simulink model "Circuit_tuner_model"  (R2022a)
settings: Solver=FixedStepAuto  StartTime=0.0  StopTime=.004  FixedStep=SampleTime  RelTol=1e-3
values from neighbouring files (symbols this model uses):
  Ad = sys_d_plasma.A    [All_injectors_LQG_bop_plasma_ss_model_code.m]    (also in All_injectors_LQG_bop_ss_model_code.m; All_injectors_LQG_continuous_time_code.m; All_injectors_LQG_plasma_7_15_24_code.m; All_injectors_LQG_plasma_ss_model_code.m)
  Amplitude = 600    [All_injectors_LQG_bop_plasma_ss_model_code.m]    (also in All_injectors_LQG_bop_ss_model_code.m; All_injectors_LQG_continuous_time_code.m; All_injectors_LQG_plasma_7_15_24_code.m; All_injectors_LQG_plasma_ss_model_code.m)
  Amplitude1 = 600    [All_injectors_vaccum.m]    (also in All_injectors_with_LQG_code.m; MPC_attempt.m; Plasma_ss_model.m; Use_for_freq_scan.m)
  Bd = sys_d_plasma.B    [All_injectors_LQG_bop_plasma_ss_model_code.m]    (also in All_injectors_LQG_bop_ss_model_code.m; All_injectors_LQG_continuous_time_code.m; All_injectors_LQG_plasma_7_15_24_code.m; All_injectors_LQG_plasma_ss_model_code.m)
  Cap = 96e-6    (= 9.6e-05)    [All_injectors_LQG_bop_ss_model_code.m]    (also in All_injectors_LQG_continuous_time_code.m; All_injectors_LQG_plasma_7_15_24_code.m; All_injectors_LQG_plasma_ss_model_code.m; All_injectors_vaccum.m)
  Cd = sys_d_plasma.C    [All_injectors_LQG_bop_plasma_ss_model_code.m]    (also in All_injectors_LQG_bop_ss_model_code.m; All_injectors_LQG_continuous_time_code.m; All_injectors_LQG_plasma_7_15_24_code.m; All_injectors_LQG_plasma_ss_model_code.m)
  Dd = sys_d_plasma.D    [All_injectors_LQG_bop_plasma_ss_model_code.m]    (also in All_injectors_LQG_bop_ss_model_code.m; All_injectors_LQG_continuous_time_code.m; All_injectors_LQG_plasma_7_15_24_code.m; All_injectors_LQG_plasma_ss_model_code.m)
  L1 = (9.78e-7)    (= 9.78e-07)    [All_injectors_LQG_bop_plasma_ss_model_code.m]    (also in All_injectors_LQG_bop_ss_model_code.m = 8.0141e-07; All_injectors_LQG_continuous_time_code.m = 8.0141e-07; All_injectors_LQG_plasma_7_15_24_code.m = 8.0141e-07; All_injectors_LQG_plasma_ss_model_code.m = 8.0141e-07)
  L2 = 2.0462e-6    (= 2.0462e-06)    [All_injectors_LQG_bop_ss_model_code.m]    (also in All_injectors_LQG_continuous_time_code.m; All_injectors_LQG_plasma_7_15_24_code.m; All_injectors_LQG_plasma_ss_model_code.m; All_injectors_vaccum.m)
  Lp = L2    (= 2.0462e-06)    [All_injectors_LQG_bop_ss_model_code.m]    (also in All_injectors_LQG_continuous_time_code.m; All_injectors_LQG_plasma_7_15_24_code.m; All_injectors_LQG_plasma_ss_model_code.m; Plasma_ss_model.m = 1.0231e-06)
  M = .161*L2    (= 3.294382e-07)    [All_injectors_LQG_bop_ss_model_code.m]    (also in All_injectors_LQG_continuous_time_code.m; All_injectors_LQG_plasma_7_15_24_code.m; All_injectors_LQG_plasma_ss_model_code.m; All_injectors_vaccum.m)
  Mw = .1346*L2    (= 2.7541852e-07)    [All_injectors_LQG_bop_ss_model_code.m]    (also in All_injectors_LQG_continuous_time_code.m; All_injectors_LQG_plasma_7_15_24_code.m; All_injectors_LQG_plasma_ss_model_code.m; All_injectors_vaccum.m)
  NoisePower = 0    [All_injectors_LQG_bop_plasma_ss_model_code.m]    (also in All_injectors_LQG_bop_ss_model_code.m = 0.0001; All_injectors_LQG_continuous_time_code.m = 0.0001; All_injectors_LQG_plasma_7_15_24_code.m; All_injectors_LQG_plasma_ss_model_code.m = 0.0001)
  R = 1    [All_injectors_LQG_bop_plasma_ss_model_code.m]    (also in All_injectors_LQG_bop_ss_model_code.m = diag(1*ones(1,num_inputs)); All_injectors_LQG_continuous_time_code.m = diag(1*ones(1,num_inputs)); All_injectors_LQG_plasma_7_15_24_code.m = diag(1*ones(1,num_inputs)); All_injectors_LQG_plasma_ss_model_code.m = diag(1*ones(1,num_inputs)))
  R1 = .0025    (= 0.0025)    [All_injectors_LQG_bop_ss_model_code.m]    (also in All_injectors_LQG_continuous_time_code.m; All_injectors_LQG_plasma_7_15_24_code.m; All_injectors_LQG_plasma_ss_model_code.m; All_injectors_vaccum.m)
  R2 = .005    (= 0.005)    [All_injectors_LQG_bop_ss_model_code.m]    (also in All_injectors_LQG_continuous_time_code.m; All_injectors_LQG_plasma_7_15_24_code.m; All_injectors_LQG_plasma_ss_model_code.m; All_injectors_vaccum.m)
  R3 = .005    (= 0.005)    [All_injectors_LQG_bop_ss_model_code.m]    (also in All_injectors_LQG_continuous_time_code.m; All_injectors_LQG_plasma_7_15_24_code.m; All_injectors_LQG_plasma_ss_model_code.m; All_injectors_vaccum.m)
  RunTime = .004    (= 0.004)    [All_injectors_LQG_bop_plasma_ss_model_code.m]    (also in All_injectors_LQG_bop_ss_model_code.m; All_injectors_LQG_continuous_time_code.m; All_injectors_LQG_plasma_7_15_24_code.m; All_injectors_LQG_plasma_ss_model_code.m)
  SampleTime = 1e-7    (= 1e-07)    [All_injectors_LQG_bop_plasma_ss_model_code.m]    (also in All_injectors_LQG_bop_ss_model_code.m; All_injectors_LQG_continuous_time_code.m; All_injectors_LQG_plasma_7_15_24_code.m; All_injectors_LQG_plasma_ss_model_code.m)
  voltage = Amplitude*sin(2*pi*Frequency*time)    [All_injectors_LQG_bop_plasma_ss_model_code.m]    (also in All_injectors_LQG_bop_ss_model_code.m; All_injectors_LQG_continuous_time_code.m; All_injectors_LQG_plasma_7_15_24_code.m; All_injectors_LQG_plasma_ss_model_code.m)
undefined symbols (not defined in the file or in its folder): Discrete, L1_V, Time
libraries: spsSeriesRLCBranchLib x49, simulink x22, spsCurrentMeasurementLib x20, spsVoltageMeasurementLib x14, spsDCVoltageSourceLib x12, spsFullBridgeMMCExternalDCLinksLib x9, spsPWMGeneratorMultilevelLib x9, spsParallelRLCBranchLib x6, ctrlSharedLib x5, spsMosfetLib x4, spsControlledVoltageSourceLib x1, spsMutualInductanceLib x1
(part 1 of 2)
settings Model: Creator=ducks  LastModifiedBy=ducks
settings DataIOCC: ExternalInput=[t,V]

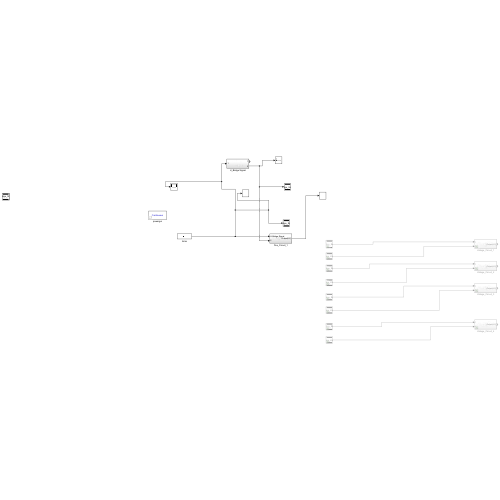
[thumbnail: Simulink's stored preview of the top-level diagram]
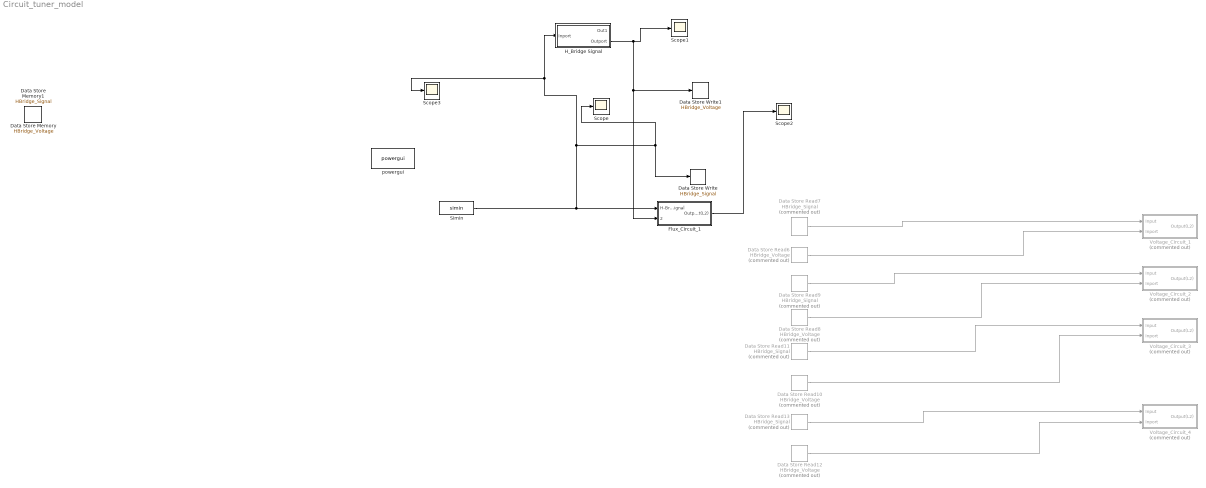
== system Circuit_tuner_model ==
  Data Store Read{6,8,10,12} (4 alike) : DataStoreRead  Commented=on  DataStoreName=HBridge_Voltage  IndexOptions=Index vector (dialog)  Indices=1  OutputSizes=1
  Data Store Read{7,9,11,13} (4 alike) : DataStoreRead  Commented=on  DataStoreName=HBridge_Signal  IndexOptions=Index vector (dialog)  Indices=1  OutputSizes=1
  Data Store Write : DataStoreWrite  DataStoreName=HBridge_Signal  IndexOptions=Index vector (dialog)  Indices=1  OutputSizes=1
  Data Store Write1 : DataStoreWrite  DataStoreName=HBridge_Voltage  IndexOptions=Index vector (dialog)  Indices=1  OutputSizes=1
  Data Store Memory : DataStoreMemory  DataStoreName=HBridge_Voltage  WriteAfterWriteMsg=warning  ShowAdditionalParam=off
  Data Store Memory1 : DataStoreMemory  DataStoreName=HBridge_Signal  WriteAfterWriteMsg=warning  ShowAdditionalParam=off
  Flux_Circuit_1 : Subsystem
  H_Bridge Signal : Subsystem
  Scope{,1..3} (4 alike) : Scope
  Simin : FromWorkspace  VariableName=simin
  Voltage_Circuit_1 : Subsystem  Commented=on
  Voltage_Circuit_2 : Subsystem  Commented=on
  Voltage_Circuit_3 : Subsystem  Commented=on
  Voltage_Circuit_4 : Subsystem  Commented=on
  powergui : spspowerguiLib/powergui  Priority=1  SimulationMode=Continuous  SampleTime=50e-6  frequency=60  Iterations=50  frequencyindice=0  Pbase=100e6  ErrMax=1e-4  UnitsV=kV  UnitsW=MW  buscounter=0  FunctionMessages=off  echomessages=off  EnableUseOfTLC=off  CurrentSourceSwitches=off  DisableSnubberDevices=off  DisableRonSwitches=off  DisableVfSwitches=off  DisplayEquations=off  AutomaticDiscreteSolvers=off  SolverType=Tustin/Backward Euler (TBE)  Interpol=off  ExternalGateDelay=off  methode=off  Ts=100  x0status=blocks  SPID=on  SwTol=0  HookPort=off  NonlinearTolerance=1e-4  nMaxIteration=100  ContinueOnMaxIteration=off  RestoreLinks=warning  ResistiveCurrentMeasurement=off  Frange=[0:2:500]  Ylog=off  Xlog=on  ShowGrid=off  save=off  variable=ZData  structure=0  ZoomFFT=off  StartTime=0.0  cycles=1  DisplayStyle=1  fundamental=60  FreqAxis=off  MaxFrequency=1000  frequencyindicesteady=1  RmsSteady=1  display=off
  wires:
  Flux_Circuit_1/1(Output(L2)) -> Scope2/1
  H_Bridge Signal/2(Outport) -> Data Store Write1/1, Flux_Circuit_1/2(2), Scope1/1
  Simin/1 -> Scope3/1, H_Bridge Signal/1(Inport), Scope/1, Data Store Write/1, Flux_Circuit_1/1(H-Bridge Signal)
  Data Store Read6/1 -> Voltage_Circuit_1/2(Inport)
  Data Store Read7/1 -> Voltage_Circuit_1/1(Input)
  Data Store Read8/1 -> Voltage_Circuit_2/2(Inport)
  Data Store Read9/1 -> Voltage_Circuit_2/1(Input)
  Data Store Read10/1 -> Voltage_Circuit_3/2(Inport)
  Data Store Read11/1 -> Voltage_Circuit_3/1(Input)
  Data Store Read12/1 -> Voltage_Circuit_4/2(Inport)
  Data Store Read13/1 -> Voltage_Circuit_4/1(Input)

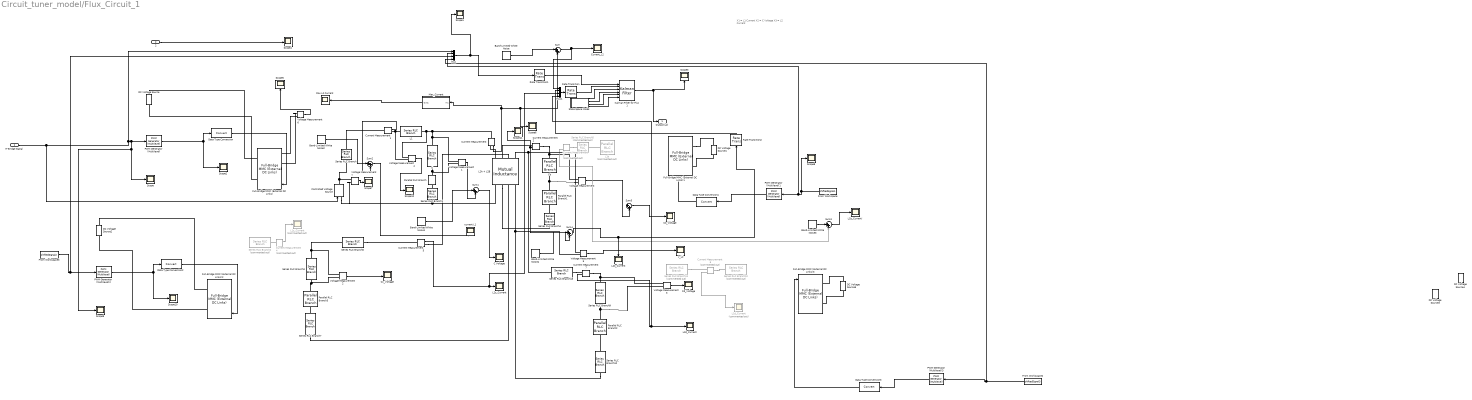
== system Circuit_tuner_model/Flux_Circuit_1 ==
  note: X1 = L1 Current
      | X2 = C Voltage
      | X3 = L2 Current
  H-Bridge Signal : Inport
  2 : Inport  Port=2
  Band-Limited White Noise{,2..4} (4 alike) : simulink/Sources/Band-Limited White Noise  Cov=NoisePower  Ts=SampleTime  seed=[23341]
  Band-Limited White Noise1 : simulink/Sources/Band-Limited White Noise  Cov=NoisePower/5  Ts=SampleTime  seed=[23341]
  C : spsSeriesRLCBranchLib/Series RLC Branch  LConnTagsString=__new0  RConnTagsString=__new0  BranchType=C  Resistance=1  Inductance=1e-3  SetiL0=off  InitialCurrent=0  Capacitance=Cap  Setx0=off  InitialVoltage=0  Measurements=None
  C Voltage : Scope
  Cb : spsParallelRLCBranchLib/Parallel RLC Branch  LConnTagsString=a  RConnTagsString=__new0  BranchType=C  Resistance=1  Inductance=1e-3  SetiL0=off  InitialCurrent=0  Capacitance=Cap  Setx0=off  InitialVoltage=0  Measurements=None
  Cb_Voltage : Scope
  Cc_Voltage : Scope
  Cd_Voltage : Scope
  Controlled Voltage Source : spsControlledVoltageSourceLib/Controlled Voltage Source  Initialize=on  Source_Type=AC  Amplitude=0  Phase=0  Frequency=0  Measurements=None
  Current Measurement{,1..2,5,7} (5 alike) : spsCurrentMeasurementLib/Current Measurement  PhasorSimulation=off  OutputType=Complex  PSBequivalent=0
  Current Measurement3 : spsCurrentMeasurementLib/Current Measurement  Commented=on  PhasorSimulation=off  OutputType=Complex  PSBequivalent=0
  Current Measurement4 : spsCurrentMeasurementLib/Current Measurement  Commented=on  PhasorSimulation=off  OutputType=Complex  PSBequivalent=0
  Current Measurement6 : spsCurrentMeasurementLib/Current Measurement  Commented=on  PhasorSimulation=off  OutputType=Complex  PSBequivalent=0
  Current_L2 : Scope
  DC Voltage Source : spsDCVoltageSourceLib/DC Voltage Source  Amplitude=Amplitude  Measurements=None
  DC Voltage Source1 : spsDCVoltageSourceLib/DC Voltage Source  Amplitude=Amplitude1  Measurements=None
  DC Voltage Source2 : spsDCVoltageSourceLib/DC Voltage Source  Amplitude=Amplitude1  Measurements=None
  DC Voltage Source3 : spsDCVoltageSourceLib/DC Voltage Source  Amplitude=Amplitude  Measurements=None
  DC Voltage Source4 : spsDCVoltageSourceLib/DC Voltage Source  Amplitude=Amplitude  Measurements=None
  DC Voltage Source5 : spsDCVoltageSourceLib/DC Voltage Source  Amplitude=Amplitude1  Measurements=None
  Data Type Conversion{,1..3} (4 alike) : DataTypeConversion  SaturateOnIntegerOverflow=off  RndMeth=Floor
  From Workspace : FromWorkspace  VariableName=shiftedSignal1
  From Workspace2 : FromWorkspace  VariableName=shiftedSignal3
  From Workspace3 : FromWorkspace  VariableName=shiftedSignal2
  Full-Bridge MMC (External DC Links){,1..3} (4 alike) : spsFullBridgeMMCExternalDCLinksLib/Full-Bridge MMC (External DC Links)  ModelType=Switching devices  n=1  Ron=1e-3  Rs=1e6  Cs=inf  Ron_Diode=1e-3  Rs_Diode=1e6  Cs_Diode=inf  Vf_Diode=1e-3  Rs_CurrentSource=inf  Ts=1e-6
      settings: SourceProductBaseCode=PS
  Kalman Filter for Flux 1 : ctrlSharedLib/Kalman Filter  TimeDomain=Discrete-Time  UseCurrentEstimator=on  ModelSource=Input port  ModelSourceVariable=sys_d  A=Ad  B=Bd  C=Cd  D=Dd  NumberOfStates=12  NumberOfInputs=4  NumberOfOutputs=4  InitialEstimateSource=Dialog  X0=voltage(1)  P0=10  UseK=off  UseGH=off  NumberOfProcessNoiseInputs=1  G=G  TimeInvariantG=on  H=0  TimeInvariantH=on  Q=Q  TimeInvariantQ=on  R=R  TimeInvariantR=on  N=0  TimeInvariantN=on  AddInputPort=on  AddEnablePort=off  OutputEstimatedY=off  OutputP=off  Ts=SampleTime
  L1 : spsSeriesRLCBranchLib/Series RLC Branch  LConnTagsString=__new0  RConnTagsString=__new0  BranchType=L  Resistance=1  Inductance=L1  SetiL0=off  InitialCurrent=0  Capacitance=0  Setx0=off  InitialVoltage=0  Measurements=None
  L1b : spsParallelRLCBranchLib/Parallel RLC Branch  Commented=on  LConnTagsString=a  RConnTagsString=__new0  BranchType=L  Resistance=1  Inductance=L1  SetiL0=off  InitialCurrent=0  Capacitance=1e-6  Setx0=off  InitialVoltage=0  Measurements=None
  L1b_Current' : Scope
  L1c_Current : Scope  Commented=on
  L1d_Current : Scope  Commented=on
  L2A + L2B : spsMutualInductanceLib/Mutual Inductance  LConnTagsString=a|b|c|L4  RConnTagsString=A|B|C|R4  TypeOfMutual=Generalized mutual inductance  NumberOfWindings=4  SelfImpedance1=[R3 L2]  SelfImpedance2=[R3 L2]  ThreeWindings=on  SelfImpedance3=[ 1.1 1.1e-03]  MutualImpedance=[R3/2 L2/2]  InductanceMatrix=[L2 M M Mw; M L2 Mw M; M Mw L2 M; Mw M M L2;]  ResistanceMatrix=[R3 0 0 0; 0 R3 0 0; 0 0 R3 0; 0 0 0 R3;]  Measurements=Winding voltages and currents
      settings: SourceProductBaseCode=PS
  L2b_Current : Scope
  L2c_Current : Scope
  L2d_Current : Scope
  Max L2 Current : Scope
  Max_Current : Subsystem
  Mux : Mux
  Mux1 : Mux
  PWM Generator (Multilevel){,1..3} (4 alike) : spsPWMGeneratorMultilevelLib/PWM Generator (Multilevel)  BridgeType=Full-bridge  NumberOfBridges=1  Fc=1e3  Ts=0  ShowCarriersOutport=off
      settings: SourceProductBaseCode=PS
  Parallel RLC Branch{,1..3} (4 alike) : spsParallelRLCBranchLib/Parallel RLC Branch  LConnTagsString=a  RConnTagsString=__new0  BranchType=L  Resistance=1  Inductance=100e-9  SetiL0=off  InitialCurrent=0  Capacitance=1e-6  Setx0=off  InitialVoltage=0  Measurements=None
  Rate Transition : RateTransition
  Rate Transition1 : RateTransition
  Rate Transition2 : RateTransition
  Scope{,1..12} (13 alike) : Scope
  Series RLC Branch : spsSeriesRLCBranchLib/Series RLC Branch  LConnTagsString=__new0  RConnTagsString=__new0  BranchType=R  Resistance=R1  Inductance=1e-3  SetiL0=off  InitialCurrent=0  Capacitance=1e-6  Setx0=off  InitialVoltage=0  Measurements=None
  Series RLC Branch{1,4,7,12} (4 alike) : spsSeriesRLCBranchLib/Series RLC Branch  LConnTagsString=__new0  RConnTagsString=__new0  BranchType=R  Resistance=R2  Inductance=1e-3  SetiL0=off  InitialCurrent=0  Capacitance=1e-6  Setx0=off  InitialVoltage=0  Measurements=None
  Series RLC Branch10 : spsSeriesRLCBranchLib/Series RLC Branch  Commented=on  LConnTagsString=__new0  RConnTagsString=__new0  BranchType=L  Resistance=1  Inductance=L1  SetiL0=off  InitialCurrent=0  Capacitance=1e-6  Setx0=off  InitialVoltage=0  Measurements=None
  Series RLC Branch11 : spsSeriesRLCBranchLib/Series RLC Branch  Commented=on  LConnTagsString=__new0  RConnTagsString=__new0  BranchType=R  Resistance=R1  Inductance=1e-3  SetiL0=off  InitialCurrent=0  Capacitance=1e-6  Setx0=off  InitialVoltage=0  Measurements=None
  Series RLC Branch13 : spsSeriesRLCBranchLib/Series RLC Branch  LConnTagsString=__new0  RConnTagsString=__new0  BranchType=R  Resistance=R3  Inductance=1e-3  SetiL0=off  InitialCurrent=0  Capacitance=1e-6  Setx0=off  InitialVoltage=0  Measurements=None
  Series RLC Branch2 : spsSeriesRLCBranchLib/Series RLC Branch  Commented=on  LConnTagsString=__new0  RConnTagsString=__new0  BranchType=L  Resistance=1  Inductance=L1  SetiL0=off  InitialCurrent=0  Capacitance=1e-6  Setx0=off  InitialVoltage=0  Measurements=None
  Series RLC Branch3 : spsSeriesRLCBranchLib/Series RLC Branch  LConnTagsString=__new0  RConnTagsString=__new0  BranchType=C  Resistance=1  Inductance=L2  SetiL0=off  InitialCurrent=0  Capacitance=Cap  Setx0=off  InitialVoltage=0  Measurements=None
  Series RLC Branch5 : spsSeriesRLCBranchLib/Series RLC Branch  Commented=on  LConnTagsString=__new0  RConnTagsString=__new0  BranchType=R  Resistance=R1  Inductance=1e-3  SetiL0=off  InitialCurrent=0  Capacitance=1e-6  Setx0=off  InitialVoltage=0  Measurements=None
  Series RLC Branch6 : spsSeriesRLCBranchLib/Series RLC Branch  LConnTagsString=__new0  RConnTagsString=__new0  BranchType=R  Resistance=R3  Inductance=1e-3  SetiL0=off  InitialCurrent=0  Capacitance=1e-6  Setx0=off  InitialVoltage=0  Measurements=None
  Series RLC Branch9 : spsSeriesRLCBranchLib/Series RLC Branch  LConnTagsString=__new0  RConnTagsString=__new0  BranchType=C  Resistance=1  Inductance=1e-3  SetiL0=off  InitialCurrent=0  Capacitance=Cap  Setx0=off  InitialVoltage=0  Measurements=None
  State Space Model : Subsystem
  Sum{,1..5} (6 alike) : Sum  Inputs=|++
  Voltage Measurement{,1..7} (8 alike) : spsVoltageMeasurementLib/Voltage Measurement  PhasorSimulation=off  OutputType=Complex  PSBequivalent=0
  current L1 : Scope
  v_L2 : Scope
  Output(L2) : Outport
  wires:
  Current Measurement1/1 -> Sum2/2
  PWM Generator (Multilevel)/1 -> Data Type Conversion/1, Scope2/1
  Band-Limited White Noise/1 -> Sum/1
  Current Measurement/1 -> Max_Current/1(In1), Scope6/1, Sum/2
  Data Type Conversion/1 -> Full-Bridge MMC (External DC Links)/1
  Kalman Filter for Flux 1/1 -> Scope3/1, Output(L2)/1
  Sum2/1 -> current L1/1
  Band-Limited White Noise1/1 -> Sum1/1
  Voltage Measurement1/1 -> Sum1/2
  Band-Limited White Noise2/1 -> Sum2/1
  Sum1/1 -> C Voltage/1
  Max_Current/1(Out1) -> Max L2 Current/1
  Sum/1 -> Mux1/1, Current_L2/1
  Data Type Conversion1/1 -> Full-Bridge MMC (External DC Links)1/1
  PWM Generator (Multilevel)1/1 -> Data Type Conversion1/1
  Rate Transition1/1 -> Kalman Filter for Flux 1/1
  Voltage Measurement/1 -> Sum5/2
  2/1 -> Scope4/1
  State Space Model/1(A) -> Kalman Filter for Flux 1/3
  State Space Model/2(B) -> Kalman Filter for Flux 1/4
  State Space Model/3(C) -> Kalman Filter for Flux 1/5
  State Space Model/4(D) -> Kalman Filter for Flux 1/6
  Mux/1 -> Scope1/1, Rate Transition1/1
  Rate Transition2/1 -> Mux1/2
  Band-Limited White Noise3/1 -> Sum3/1
  Current Measurement3/1 -> Sum3/2
  Sum3/1 -> L1b_Current'/1
  Band-Limited White Noise4/1 -> Sum4/1
  Current Measurement2/1 -> Sum4/2, Scope11/1
  Sum4/1 -> Rate Transition2/1, L2b_Current/1
  Sum5/1 -> Cb_Voltage/1
  Mux1/1 -> Rate Transition/1
  From Workspace/1 -> PWM Generator (Multilevel)1/1, Mux/2, Scope8/1
  H-Bridge Signal/1 -> Controlled Voltage Source/1, Mux/1, Scope9/1, Scope/1, PWM Generator (Multilevel)/1
  Data Type Conversion2/1 -> Full-Bridge MMC (External DC Links)2/1
  PWM Generator (Multilevel)2/1 -> Data Type Conversion2/1, Scope10/1
  Voltage Measurement2/1 -> Cc_Voltage/1
  Current Measurement4/1 -> L1c_Current/1
  PWM Generator (Multilevel)3/1 -> Data Type Conversion3/1
  Data Type Conversion3/1 -> Full-Bridge MMC (External DC Links)3/1
  Current Measurement5/1 -> Mux1/3, L2c_Current/1
  Voltage Measurement3/1 -> Cd_Voltage/1
  Current Measurement6/1 -> L1d_Current/1
  Current Measurement7/1 -> L2d_Current/1, Mux1/4
  Rate Transition/1 -> Kalman Filter for Flux 1/2
  From Workspace2/1 -> Mux/4, PWM Generator (Multilevel)3/1
  From Workspace3/1 -> Mux/3, PWM Generator (Multilevel)2/1
  Voltage Measurement4/1 -> Scope12/1
  Voltage Measurement5/1 -> v_L2/1
  Voltage Measurement6/1 -> Scope5/1
  Voltage Measurement7/1 -> Scope7/1
  connections:
  Current Measurement1/LConn1 -- Series RLC Branch/LConn1
  Current Measurement1/RConn1 -- Voltage Measurement4/LConn2 -- L1/LConn1
  Full-Bridge MMC (External DC Links)/RConn1 -- DC Voltage Source/RConn1
  Full-Bridge MMC (External DC Links)/RConn2 -- DC Voltage Source/LConn1
  Voltage Measurement6/LConn1 -- Full-Bridge MMC (External DC Links)/LConn1
  Voltage Measurement6/LConn2 -- Full-Bridge MMC (External DC Links)/LConn2
  L2A + L2B/LConn1 -- Current Measurement/RConn1
  L1/RConn1 -- Voltage Measurement4/LConn1 -- Current Measurement/LConn1 -- Voltage Measurement1/LConn1 -- C/LConn1
  Voltage Measurement1/LConn2 -- Parallel RLC Branch/LConn1 -- C/RConn1
  Current Measurement2/LConn1 -- Voltage Measurement/LConn1 -- Cb/LConn1
  L2A + L2B/RConn2 -- Series RLC Branch4/RConn1
  Series RLC Branch4/LConn1 -- Parallel RLC Branch1/RConn1
  L1b/LConn1 -- Series RLC Branch5/LConn1
  Full-Bridge MMC (External DC Links)1/RConn2 -- DC Voltage Source1/LConn1
  Full-Bridge MMC (External DC Links)1/RConn1 -- DC Voltage Source1/RConn1
  Current Measurement2/RConn1 -- L2A + L2B/LConn2
  Current Measurement3/LConn1 -- Series RLC Branch5/RConn1
  Voltage Measurement2/LConn1 -- Series RLC Branch6/LConn1 -- Series RLC Branch3/LConn1
  Voltage Measurement2/LConn2 -- Parallel RLC Branch3/LConn1 -- Series RLC Branch3/RConn1
  Current Measurement5/RConn1 -- L2A + L2B/LConn3
  Series RLC Branch7/RConn1 -- L2A + L2B/RConn3
  Full-Bridge MMC (External DC Links)2/RConn1 -- DC Voltage Source2/RConn1
  Full-Bridge MMC (External DC Links)2/RConn2 -- DC Voltage Source2/LConn1
  Current Measurement4/LConn1 -- Series RLC Branch2/RConn1
  Series RLC Branch6/RConn1 -- Current Measurement5/LConn1
  Current Measurement6/LConn1 -- Series RLC Branch10/LConn1
  Series RLC Branch9/LConn1 -- Current Measurement7/LConn1 -- Voltage Measurement3/LConn1
  Series RLC Branch12/LConn1 -- Parallel RLC Branch2/RConn1
  Series RLC Branch13/LConn1 -- L2A + L2B/LConn4 -- Voltage Measurement5/LConn1
  DC Voltage Source5/RConn1 -- Full-Bridge MMC (External DC Links)3/RConn1
  Full-Bridge MMC (External DC Links)3/RConn2 -- DC Voltage Source5/LConn1
  Series RLC Branch12/RConn1 -- L2A + L2B/RConn4 -- Voltage Measurement5/LConn2
  Series RLC Branch11/RConn1 -- Current Measurement6/RConn1
  Series RLC Branch13/RConn1 -- Current Measurement7/RConn1
  Series RLC Branch1/LConn1 -- Parallel RLC Branch/RConn1
  Series RLC Branch7/LConn1 -- Parallel RLC Branch3/RConn1
  Parallel RLC Branch2/LConn1 -- Voltage Measurement3/LConn2 -- Series RLC Branch9/RConn1
  Parallel RLC Branch1/LConn1 -- Cb/RConn1 -- Voltage Measurement/LConn2
  Series RLC Branch1/RConn1 -- Voltage Measurement7/LConn2 -- Controlled Voltage Source/LConn1 -- L2A + L2B/RConn1
  Controlled Voltage Source/RConn1 -- Series RLC Branch/RConn1 -- Voltage Measurement7/LConn1

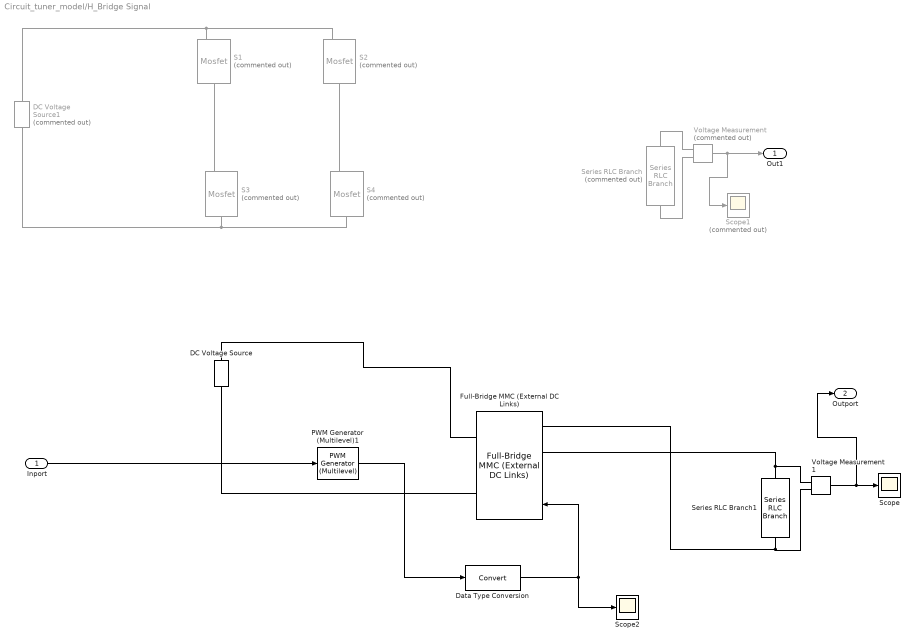
== system Circuit_tuner_model/H_Bridge Signal ==
  Inport : Inport
  DC Voltage Source : spsDCVoltageSourceLib/DC Voltage Source  Amplitude=600  Measurements=None
  DC Voltage Source1 : spsDCVoltageSourceLib/DC Voltage Source  Commented=on  Amplitude=600  Measurements=None
  Data Type Conversion : DataTypeConversion  SaturateOnIntegerOverflow=off  RndMeth=Floor
  Full-Bridge MMC (External DC Links) : spsFullBridgeMMCExternalDCLinksLib/Full-Bridge MMC (External DC Links)  ModelType=Switching devices  n=1  Ron=1e-3  Rs=1e6  Cs=inf  Ron_Diode=1e-3  Rs_Diode=1e6  Cs_Diode=inf  Vf_Diode=1e-3  Rs_CurrentSource=inf  Ts=10e-6
      settings: SourceProductBaseCode=PS
  PWM Generator (Multilevel)1 : spsPWMGeneratorMultilevelLib/PWM Generator (Multilevel)  BridgeType=Full-bridge  NumberOfBridges=1  Fc=1e3  Ts=0  ShowCarriersOutport=off
      settings: SourceProductBaseCode=PS
  S{1..4} (4 alike) : spsMosfetLib/Mosfet  Commented=on  Ron=0.1  Lon=0  Rd=0.01  Vfd=0  IC=0  Rs=1e5  Cs=inf  Measurements=off
  Scope : Scope
  Scope1 : Scope  Commented=on
  Scope2 : Scope
  Series RLC Branch : spsSeriesRLCBranchLib/Series RLC Branch  Commented=on  LConnTagsString=__new0  RConnTagsString=__new0  BranchType=R  Resistance=1  Inductance=1e-3  SetiL0=off  InitialCurrent=0  Capacitance=1e-6  Setx0=off  InitialVoltage=0  Measurements=None
  Series RLC Branch1 : spsSeriesRLCBranchLib/Series RLC Branch  LConnTagsString=__new0  RConnTagsString=__new0  BranchType=R  Resistance=1  Inductance=1e-3  SetiL0=off  InitialCurrent=0  Capacitance=1e-6  Setx0=off  InitialVoltage=0  Measurements=None
  Voltage Measurement : spsVoltageMeasurementLib/Voltage Measurement  Commented=on  PhasorSimulation=off  OutputType=Complex  PSBequivalent=0
  Voltage Measurement1 : spsVoltageMeasurementLib/Voltage Measurement  PhasorSimulation=off  OutputType=Complex  PSBequivalent=0
  Out1 : Outport
  Outport : Outport  Port=2
  wires:
  Voltage Measurement/1 -> Scope1/1, Out1/1
  PWM Generator (Multilevel)1/1 -> Data Type Conversion/1
  Inport/1 -> PWM Generator (Multilevel)1/1
  Data Type Conversion/1 -> Full-Bridge MMC (External DC Links)/1, Scope2/1
  Voltage Measurement1/1 -> Outport/1, Scope/1
  connections:
  Voltage Measurement/LConn1 -- Series RLC Branch/LConn1
  Voltage Measurement/LConn2 -- Series RLC Branch/RConn1
  S1/LConn1 -- S2/LConn1 -- DC Voltage Source1/LConn1
  S1/RConn1 -- S3/LConn1
  S3/RConn1 -- DC Voltage Source1/RConn1 -- S4/RConn1
  S4/LConn1 -- S2/RConn1
  Voltage Measurement1/LConn2 -- Full-Bridge MMC (External DC Links)/LConn2 -- Series RLC Branch1/RConn1
  Full-Bridge MMC (External DC Links)/RConn2 -- DC Voltage Source/LConn1
  Voltage Measurement1/LConn1 -- Full-Bridge MMC (External DC Links)/LConn1 -- Series RLC Branch1/LConn1
  Full-Bridge MMC (External DC Links)/RConn1 -- DC Voltage Source/RConn1

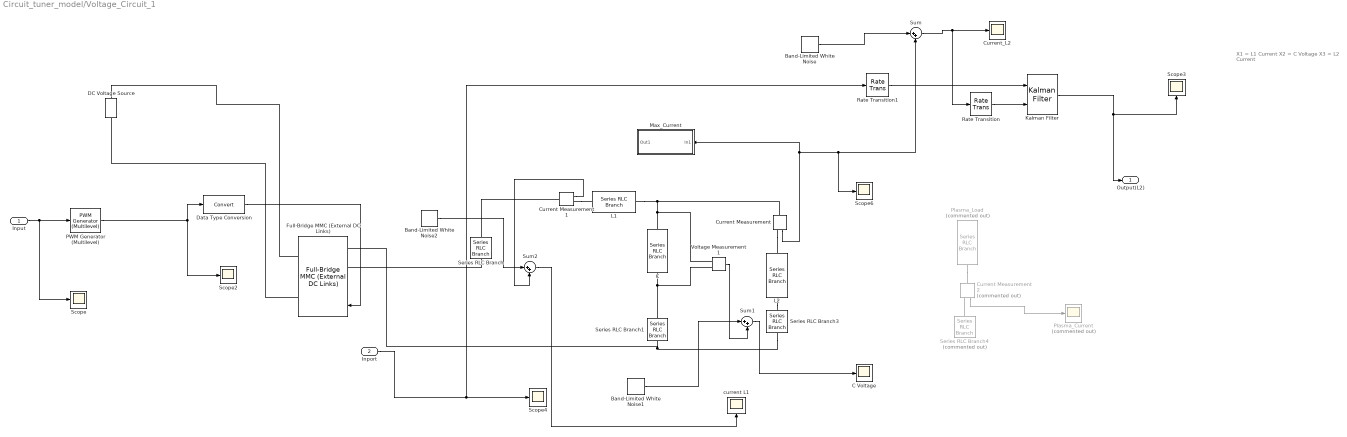
== system Circuit_tuner_model/Voltage_Circuit_1 ==
  note: X1 = L1 Current
      | X2 = C Voltage
      | X3 = L2 Current
  Input : Inport
  Inport : Inport  Port=2
  Band-Limited White Noise : simulink/Sources/Band-Limited White Noise  Cov=NoisePower  Ts=SampleTime  seed=[23341]
  Band-Limited White Noise1 : simulink/Sources/Band-Limited White Noise  Cov=NoisePower/5  Ts=SampleTime  seed=[23341]
  Band-Limited White Noise2 : simulink/Sources/Band-Limited White Noise  Cov=NoisePower  Ts=SampleTime  seed=[23341]
  C : spsSeriesRLCBranchLib/Series RLC Branch  LConnTagsString=__new0  RConnTagsString=__new0  BranchType=C  Resistance=1  Inductance=1e-3  SetiL0=off  InitialCurrent=0  Capacitance=Cap*2  Setx0=off  InitialVoltage=0  Measurements=None
  C Voltage : Scope
  Current Measurement : spsCurrentMeasurementLib/Current Measurement  PhasorSimulation=off  OutputType=Complex  PSBequivalent=0
  Current Measurement1 : spsCurrentMeasurementLib/Current Measurement  PhasorSimulation=off  OutputType=Complex  PSBequivalent=0
  Current Measurement2 : spsCurrentMeasurementLib/Current Measurement  Commented=on  PhasorSimulation=off  OutputType=Complex  PSBequivalent=0
  Current_L2 : Scope
  DC Voltage Source : spsDCVoltageSourceLib/DC Voltage Source  Amplitude=Amplitude  Measurements=None
  Data Type Conversion : DataTypeConversion  SaturateOnIntegerOverflow=off  RndMeth=Floor
  Full-Bridge MMC (External DC Links) : spsFullBridgeMMCExternalDCLinksLib/Full-Bridge MMC (External DC Links)  ModelType=Switching devices  n=1  Ron=1e-3  Rs=1e6  Cs=inf  Ron_Diode=1e-3  Rs_Diode=1e6  Cs_Diode=inf  Vf_Diode=1e-3  Rs_CurrentSource=inf  Ts=1e-6
      settings: SourceProductBaseCode=PS
  Kalman Filter : ctrlSharedLib/Kalman Filter  TimeDomain=Discrete-Time  UseCurrentEstimator=on  ModelSource=LTI State-Space Variable  ModelSourceVariable=sys_d  A=Ad  B=Bd  C=Cd  D=Dd  NumberOfStates=1  NumberOfInputs=1  NumberOfOutputs=1  InitialEstimateSource=Dialog  X0=voltage(1)  P0=10  UseK=off  UseGH=off  NumberOfProcessNoiseInputs=1  G=G  TimeInvariantG=on  H=0  TimeInvariantH=on  Q=Q  TimeInvariantQ=on  R=R  TimeInvariantR=on  N=0  TimeInvariantN=on  AddInputPort=on  AddEnablePort=off  OutputEstimatedY=off  OutputP=off  Ts=SampleTime
  L1 : spsSeriesRLCBranchLib/Series RLC Branch  LConnTagsString=__new0  RConnTagsString=__new0  BranchType=L  Resistance=1  Inductance=L1_V  SetiL0=off  InitialCurrent=0  Capacitance=0  Setx0=off  InitialVoltage=0  Measurements=None
  L2 : spsSeriesRLCBranchLib/Series RLC Branch  LConnTagsString=__new0  RConnTagsString=__new0  BranchType=L  Resistance=1  Inductance=L2  SetiL0=off  InitialCurrent=0  Capacitance=1e-6  Setx0=off  InitialVoltage=0  Measurements=None
  Max_Current : Subsystem
  PWM Generator (Multilevel) : spsPWMGeneratorMultilevelLib/PWM Generator (Multilevel)  BridgeType=Full-bridge  NumberOfBridges=1  Fc=1e3  Ts=0  ShowCarriersOutport=off
      settings: SourceProductBaseCode=PS
  Plasma_Current : Scope  Commented=on
  Plasma_Load : spsSeriesRLCBranchLib/Series RLC Branch  Commented=on  LConnTagsString=__new0  RConnTagsString=__new0  BranchType=L  Resistance=1  Inductance=Lp  SetiL0=off  InitialCurrent=0  Capacitance=1e-6  Setx0=off  InitialVoltage=0  Measurements=None
  Rate Transition : RateTransition
  Rate Transition1 : RateTransition
  Scope{,2..4,6} (5 alike) : Scope
  Series RLC Branch : spsSeriesRLCBranchLib/Series RLC Branch  LConnTagsString=__new0  RConnTagsString=__new0  BranchType=R  Resistance=R1  Inductance=1e-3  SetiL0=off  InitialCurrent=0  Capacitance=1e-6  Setx0=off  InitialVoltage=0  Measurements=None
  Series RLC Branch1 : spsSeriesRLCBranchLib/Series RLC Branch  LConnTagsString=__new0  RConnTagsString=__new0  BranchType=R  Resistance=R2  Inductance=1e-3  SetiL0=off  InitialCurrent=0  Capacitance=1e-6  Setx0=off  InitialVoltage=0  Measurements=None
  Series RLC Branch3 : spsSeriesRLCBranchLib/Series RLC Branch  LConnTagsString=__new0  RConnTagsString=__new0  BranchType=R  Resistance=R3  Inductance=1e-3  SetiL0=off  InitialCurrent=0  Capacitance=1e-6  Setx0=off  InitialVoltage=0  Measurements=None
  Series RLC Branch4 : spsSeriesRLCBranchLib/Series RLC Branch  Commented=on  LConnTagsString=__new0  RConnTagsString=__new0  BranchType=R  Resistance=.005  Inductance=1e-3  SetiL0=off  InitialCurrent=0  Capacitance=1e-6  Setx0=off  InitialVoltage=0  Measurements=None
  Sum : Sum  Inputs=|++
  Sum1 : Sum  Inputs=|++
  Sum2 : Sum  Inputs=|++
  Voltage Measurement1 : spsVoltageMeasurementLib/Voltage Measurement  PhasorSimulation=off  OutputType=Complex  PSBequivalent=0
  current L1 : Scope
  Output(L2) : Outport
  wires:
  Current Measurement1/1 -> Sum2/2
  PWM Generator (Multilevel)/1 -> Data Type Conversion/1, Scope2/1
  Input/1 -> Scope/1, PWM Generator (Multilevel)/1
  Current Measurement2/1 -> Plasma_Current/1
  Band-Limited White Noise/1 -> Sum/1
  Current Measurement/1 -> Max_Current/1(In1), Scope6/1, Sum/2
  Data Type Conversion/1 -> Full-Bridge MMC (External DC Links)/1
  Kalman Filter/1 -> Scope3/1, Output(L2)/1
  Sum2/1 -> current L1/1
  Band-Limited White Noise1/1 -> Sum1/1
  Voltage Measurement1/1 -> Sum1/2
  Band-Limited White Noise2/1 -> Sum2/1
  Sum1/1 -> C Voltage/1
  Sum/1 -> Rate Transition/1, Current_L2/1
  Inport/1 -> Rate Transition1/1, Scope4/1
  Rate Transition/1 -> Kalman Filter/2
  Rate Transition1/1 -> Kalman Filter/1
  connections:
  Current Measurement1/LConn1 -- Series RLC Branch/LConn1
  Current Measurement1/RConn1 -- L1/LConn1
  Series RLC Branch3/RConn1 -- Full-Bridge MMC (External DC Links)/LConn2 -- Series RLC Branch1/RConn1
  Full-Bridge MMC (External DC Links)/RConn1 -- DC Voltage Source/RConn1
  Full-Bridge MMC (External DC Links)/RConn2 -- DC Voltage Source/LConn1
  Series RLC Branch/RConn1 -- Full-Bridge MMC (External DC Links)/LConn1
  Plasma_Load/RConn1 -- Current Measurement2/LConn1
  Series RLC Branch4/LConn1 -- Current Measurement2/RConn1
  L2/RConn1 -- Series RLC Branch3/LConn1
  Current Measurement/RConn1 -- L2/LConn1
  L1/RConn1 -- Current Measurement/LConn1 -- Voltage Measurement1/LConn1 -- C/LConn1
  Series RLC Branch1/LConn1 -- Voltage Measurement1/LConn2 -- C/RConn1

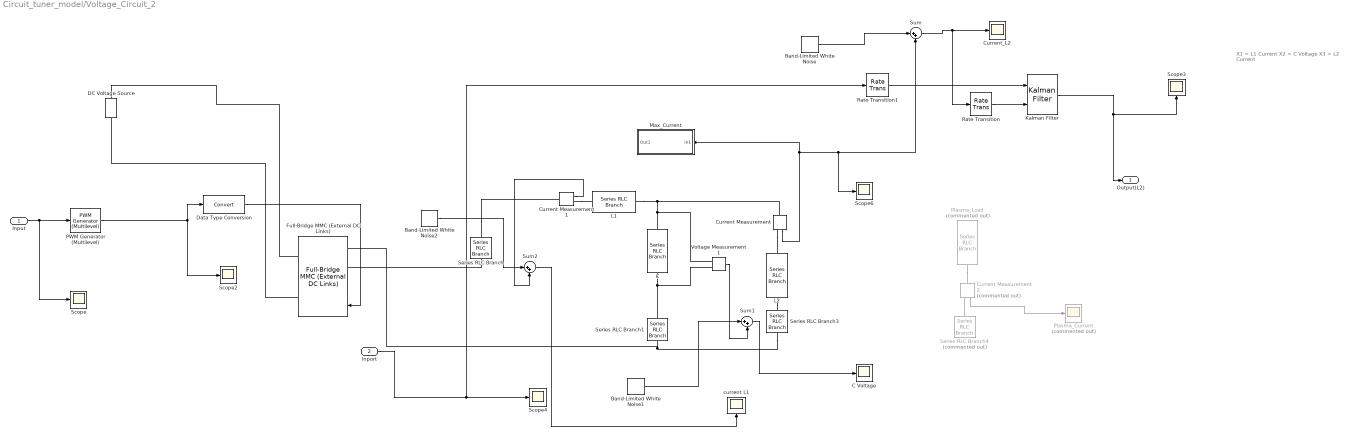
== system Circuit_tuner_model/Voltage_Circuit_2 ==
  note: X1 = L1 Current
      | X2 = C Voltage
      | X3 = L2 Current
  Input : Inport
  Inport : Inport  Port=2
  Band-Limited White Noise : simulink/Sources/Band-Limited White Noise  Cov=NoisePower  Ts=SampleTime  seed=[23341]
  Band-Limited White Noise1 : simulink/Sources/Band-Limited White Noise  Cov=NoisePower/5  Ts=SampleTime  seed=[23341]
  Band-Limited White Noise2 : simulink/Sources/Band-Limited White Noise  Cov=NoisePower  Ts=SampleTime  seed=[23341]
  C : spsSeriesRLCBranchLib/Series RLC Branch  LConnTagsString=__new0  RConnTagsString=__new0  BranchType=C  Resistance=1  Inductance=1e-3  SetiL0=off  InitialCurrent=0  Capacitance=Cap*2  Setx0=off  InitialVoltage=0  Measurements=None
  C Voltage : Scope
  Current Measurement : spsCurrentMeasurementLib/Current Measurement  PhasorSimulation=off  OutputType=Complex  PSBequivalent=0
  Current Measurement1 : spsCurrentMeasurementLib/Current Measurement  PhasorSimulation=off  OutputType=Complex  PSBequivalent=0
  Current Measurement2 : spsCurrentMeasurementLib/Current Measurement  Commented=on  PhasorSimulation=off  OutputType=Complex  PSBequivalent=0
  Current_L2 : Scope
  DC Voltage Source : spsDCVoltageSourceLib/DC Voltage Source  Amplitude=Amplitude  Measurements=None
  Data Type Conversion : DataTypeConversion  SaturateOnIntegerOverflow=off  RndMeth=Floor
  Full-Bridge MMC (External DC Links) : spsFullBridgeMMCExternalDCLinksLib/Full-Bridge MMC (External DC Links)  ModelType=Switching devices  n=1  Ron=1e-3  Rs=1e6  Cs=inf  Ron_Diode=1e-3  Rs_Diode=1e6  Cs_Diode=inf  Vf_Diode=1e-3  Rs_CurrentSource=inf  Ts=1e-6
      settings: SourceProductBaseCode=PS
  Kalman Filter : ctrlSharedLib/Kalman Filter  TimeDomain=Discrete-Time  UseCurrentEstimator=on  ModelSource=LTI State-Space Variable  ModelSourceVariable=sys_d  A=Ad  B=Bd  C=Cd  D=Dd  NumberOfStates=1  NumberOfInputs=1  NumberOfOutputs=1  InitialEstimateSource=Dialog  X0=voltage(1)  P0=10  UseK=off  UseGH=off  NumberOfProcessNoiseInputs=1  G=G  TimeInvariantG=on  H=0  TimeInvariantH=on  Q=Q  TimeInvariantQ=on  R=R  TimeInvariantR=on  N=0  TimeInvariantN=on  AddInputPort=on  AddEnablePort=off  OutputEstimatedY=off  OutputP=off  Ts=SampleTime
  L1 : spsSeriesRLCBranchLib/Series RLC Branch  LConnTagsString=__new0  RConnTagsString=__new0  BranchType=L  Resistance=1  Inductance=L1_V  SetiL0=off  InitialCurrent=0  Capacitance=0  Setx0=off  InitialVoltage=0  Measurements=None
  L2 : spsSeriesRLCBranchLib/Series RLC Branch  LConnTagsString=__new0  RConnTagsString=__new0  BranchType=L  Resistance=1  Inductance=L2  SetiL0=off  InitialCurrent=0  Capacitance=1e-6  Setx0=off  InitialVoltage=0  Measurements=None
  Max_Current : Subsystem
  PWM Generator (Multilevel) : spsPWMGeneratorMultilevelLib/PWM Generator (Multilevel)  BridgeType=Full-bridge  NumberOfBridges=1  Fc=1e3  Ts=0  ShowCarriersOutport=off
      settings: SourceProductBaseCode=PS
  Plasma_Current : Scope  Commented=on
  Plasma_Load : spsSeriesRLCBranchLib/Series RLC Branch  Commented=on  LConnTagsString=__new0  RConnTagsString=__new0  BranchType=L  Resistance=1  Inductance=Lp  SetiL0=off  InitialCurrent=0  Capacitance=1e-6  Setx0=off  InitialVoltage=0  Measurements=None
  Rate Transition : RateTransition
  Rate Transition1 : RateTransition
  Scope{,2..4,6} (5 alike) : Scope
  Series RLC Branch : spsSeriesRLCBranchLib/Series RLC Branch  LConnTagsString=__new0  RConnTagsString=__new0  BranchType=R  Resistance=R1  Inductance=1e-3  SetiL0=off  InitialCurrent=0  Capacitance=1e-6  Setx0=off  InitialVoltage=0  Measurements=None
  Series RLC Branch1 : spsSeriesRLCBranchLib/Series RLC Branch  LConnTagsString=__new0  RConnTagsString=__new0  BranchType=R  Resistance=R2  Inductance=1e-3  SetiL0=off  InitialCurrent=0  Capacitance=1e-6  Setx0=off  InitialVoltage=0  Measurements=None
  Series RLC Branch3 : spsSeriesRLCBranchLib/Series RLC Branch  LConnTagsString=__new0  RConnTagsString=__new0  BranchType=R  Resistance=R3  Inductance=1e-3  SetiL0=off  InitialCurrent=0  Capacitance=1e-6  Setx0=off  InitialVoltage=0  Measurements=None
  Series RLC Branch4 : spsSeriesRLCBranchLib/Series RLC Branch  Commented=on  LConnTagsString=__new0  RConnTagsString=__new0  BranchType=R  Resistance=.005  Inductance=1e-3  SetiL0=off  InitialCurrent=0  Capacitance=1e-6  Setx0=off  InitialVoltage=0  Measurements=None
  Sum : Sum  Inputs=|++
  Sum1 : Sum  Inputs=|++
  Sum2 : Sum  Inputs=|++
  Voltage Measurement1 : spsVoltageMeasurementLib/Voltage Measurement  PhasorSimulation=off  OutputType=Complex  PSBequivalent=0
  current L1 : Scope
  Output(L2) : Outport
  wires:
  Current Measurement1/1 -> Sum2/2
  PWM Generator (Multilevel)/1 -> Data Type Conversion/1, Scope2/1
  Input/1 -> Scope/1, PWM Generator (Multilevel)/1
  Current Measurement2/1 -> Plasma_Current/1
  Band-Limited White Noise/1 -> Sum/1
  Current Measurement/1 -> Max_Current/1(In1), Scope6/1, Sum/2
  Data Type Conversion/1 -> Full-Bridge MMC (External DC Links)/1
  Kalman Filter/1 -> Scope3/1, Output(L2)/1
  Sum2/1 -> current L1/1
  Band-Limited White Noise1/1 -> Sum1/1
  Voltage Measurement1/1 -> Sum1/2
  Band-Limited White Noise2/1 -> Sum2/1
  Sum1/1 -> C Voltage/1
  Sum/1 -> Rate Transition/1, Current_L2/1
  Inport/1 -> Rate Transition1/1, Scope4/1
  Rate Transition/1 -> Kalman Filter/2
  Rate Transition1/1 -> Kalman Filter/1
  connections:
  Current Measurement1/LConn1 -- Series RLC Branch/LConn1
  Current Measurement1/RConn1 -- L1/LConn1
  Series RLC Branch3/RConn1 -- Full-Bridge MMC (External DC Links)/LConn2 -- Series RLC Branch1/RConn1
  Full-Bridge MMC (External DC Links)/RConn1 -- DC Voltage Source/RConn1
  Full-Bridge MMC (External DC Links)/RConn2 -- DC Voltage Source/LConn1
  Series RLC Branch/RConn1 -- Full-Bridge MMC (External DC Links)/LConn1
  Plasma_Load/RConn1 -- Current Measurement2/LConn1
  Series RLC Branch4/LConn1 -- Current Measurement2/RConn1
  L2/RConn1 -- Series RLC Branch3/LConn1
  Current Measurement/RConn1 -- L2/LConn1
  L1/RConn1 -- Current Measurement/LConn1 -- Voltage Measurement1/LConn1 -- C/LConn1
  Series RLC Branch1/LConn1 -- Voltage Measurement1/LConn2 -- C/RConn1

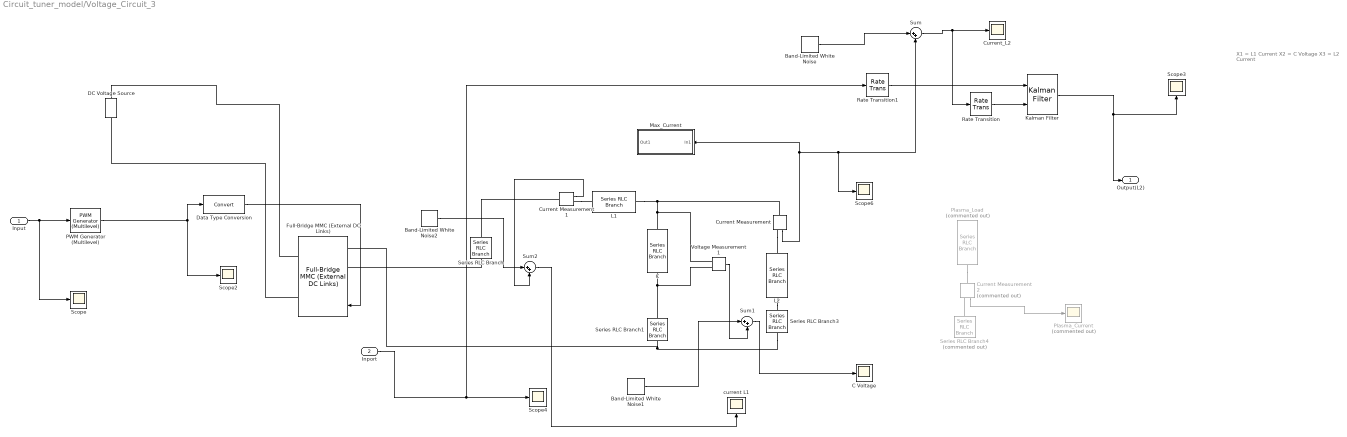
== system Circuit_tuner_model/Voltage_Circuit_3 ==
  note: X1 = L1 Current
      | X2 = C Voltage
      | X3 = L2 Current
  Input : Inport
  Inport : Inport  Port=2
  Band-Limited White Noise : simulink/Sources/Band-Limited White Noise  Cov=NoisePower  Ts=SampleTime  seed=[23341]
  Band-Limited White Noise1 : simulink/Sources/Band-Limited White Noise  Cov=NoisePower/5  Ts=SampleTime  seed=[23341]
  Band-Limited White Noise2 : simulink/Sources/Band-Limited White Noise  Cov=NoisePower  Ts=SampleTime  seed=[23341]
  C : spsSeriesRLCBranchLib/Series RLC Branch  LConnTagsString=__new0  RConnTagsString=__new0  BranchType=C  Resistance=1  Inductance=1e-3  SetiL0=off  InitialCurrent=0  Capacitance=Cap*2  Setx0=off  InitialVoltage=0  Measurements=None
  C Voltage : Scope
  Current Measurement : spsCurrentMeasurementLib/Current Measurement  PhasorSimulation=off  OutputType=Complex  PSBequivalent=0
  Current Measurement1 : spsCurrentMeasurementLib/Current Measurement  PhasorSimulation=off  OutputType=Complex  PSBequivalent=0
  Current Measurement2 : spsCurrentMeasurementLib/Current Measurement  Commented=on  PhasorSimulation=off  OutputType=Complex  PSBequivalent=0
  Current_L2 : Scope
  DC Voltage Source : spsDCVoltageSourceLib/DC Voltage Source  Amplitude=Amplitude  Measurements=None
  Data Type Conversion : DataTypeConversion  SaturateOnIntegerOverflow=off  RndMeth=Floor
  Full-Bridge MMC (External DC Links) : spsFullBridgeMMCExternalDCLinksLib/Full-Bridge MMC (External DC Links)  ModelType=Switching devices  n=1  Ron=1e-3  Rs=1e6  Cs=inf  Ron_Diode=1e-3  Rs_Diode=1e6  Cs_Diode=inf  Vf_Diode=1e-3  Rs_CurrentSource=inf  Ts=1e-6
      settings: SourceProductBaseCode=PS
  Kalman Filter : ctrlSharedLib/Kalman Filter  TimeDomain=Discrete-Time  UseCurrentEstimator=on  ModelSource=LTI State-Space Variable  ModelSourceVariable=sys_d  A=Ad  B=Bd  C=Cd  D=Dd  NumberOfStates=1  NumberOfInputs=1  NumberOfOutputs=1  InitialEstimateSource=Dialog  X0=voltage(1)  P0=10  UseK=off  UseGH=off  NumberOfProcessNoiseInputs=1  G=G  TimeInvariantG=on  H=0  TimeInvariantH=on  Q=Q  TimeInvariantQ=on  R=R  TimeInvariantR=on  N=0  TimeInvariantN=on  AddInputPort=on  AddEnablePort=off  OutputEstimatedY=off  OutputP=off  Ts=SampleTime
  L1 : spsSeriesRLCBranchLib/Series RLC Branch  LConnTagsString=__new0  RConnTagsString=__new0  BranchType=L  Resistance=1  Inductance=L1_V  SetiL0=off  InitialCurrent=0  Capacitance=0  Setx0=off  InitialVoltage=0  Measurements=None
  L2 : spsSeriesRLCBranchLib/Series RLC Branch  LConnTagsString=__new0  RConnTagsString=__new0  BranchType=L  Resistance=1  Inductance=L2  SetiL0=off  InitialCurrent=0  Capacitance=1e-6  Setx0=off  InitialVoltage=0  Measurements=None
  Max_Current : Subsystem
  PWM Generator (Multilevel) : spsPWMGeneratorMultilevelLib/PWM Generator (Multilevel)  BridgeType=Full-bridge  NumberOfBridges=1  Fc=1e3  Ts=0  ShowCarriersOutport=off
      settings: SourceProductBaseCode=PS
  Plasma_Current : Scope  Commented=on
  Plasma_Load : spsSeriesRLCBranchLib/Series RLC Branch  Commented=on  LConnTagsString=__new0  RConnTagsString=__new0  BranchType=L  Resistance=1  Inductance=Lp  SetiL0=off  InitialCurrent=0  Capacitance=1e-6  Setx0=off  InitialVoltage=0  Measurements=None
  Rate Transition : RateTransition
  Rate Transition1 : RateTransition
  Scope{,2..4,6} (5 alike) : Scope
  Series RLC Branch : spsSeriesRLCBranchLib/Series RLC Branch  LConnTagsString=__new0  RConnTagsString=__new0  BranchType=R  Resistance=R1  Inductance=1e-3  SetiL0=off  InitialCurrent=0  Capacitance=1e-6  Setx0=off  InitialVoltage=0  Measurements=None
  Series RLC Branch1 : spsSeriesRLCBranchLib/Series RLC Branch  LConnTagsString=__new0  RConnTagsString=__new0  BranchType=R  Resistance=R2  Inductance=1e-3  SetiL0=off  InitialCurrent=0  Capacitance=1e-6  Setx0=off  InitialVoltage=0  Measurements=None
  Series RLC Branch3 : spsSeriesRLCBranchLib/Series RLC Branch  LConnTagsString=__new0  RConnTagsString=__new0  BranchType=R  Resistance=R3  Inductance=1e-3  SetiL0=off  InitialCurrent=0  Capacitance=1e-6  Setx0=off  InitialVoltage=0  Measurements=None
  Series RLC Branch4 : spsSeriesRLCBranchLib/Series RLC Branch  Commented=on  LConnTagsString=__new0  RConnTagsString=__new0  BranchType=R  Resistance=.005  Inductance=1e-3  SetiL0=off  InitialCurrent=0  Capacitance=1e-6  Setx0=off  InitialVoltage=0  Measurements=None
  Sum : Sum  Inputs=|++
  Sum1 : Sum  Inputs=|++
  Sum2 : Sum  Inputs=|++
  Voltage Measurement1 : spsVoltageMeasurementLib/Voltage Measurement  PhasorSimulation=off  OutputType=Complex  PSBequivalent=0
  current L1 : Scope
  Output(L2) : Outport
  wires:
  Current Measurement1/1 -> Sum2/2
  PWM Generator (Multilevel)/1 -> Data Type Conversion/1, Scope2/1
  Input/1 -> Scope/1, PWM Generator (Multilevel)/1
  Current Measurement2/1 -> Plasma_Current/1
  Band-Limited White Noise/1 -> Sum/1
  Current Measurement/1 -> Max_Current/1(In1), Scope6/1, Sum/2
  Data Type Conversion/1 -> Full-Bridge MMC (External DC Links)/1
  Kalman Filter/1 -> Scope3/1, Output(L2)/1
  Sum2/1 -> current L1/1
  Band-Limited White Noise1/1 -> Sum1/1
  Voltage Measurement1/1 -> Sum1/2
  Band-Limited White Noise2/1 -> Sum2/1
  Sum1/1 -> C Voltage/1
  Sum/1 -> Rate Transition/1, Current_L2/1
  Inport/1 -> Rate Transition1/1, Scope4/1
  Rate Transition/1 -> Kalman Filter/2
  Rate Transition1/1 -> Kalman Filter/1
  connections:
  Current Measurement1/LConn1 -- Series RLC Branch/LConn1
  Current Measurement1/RConn1 -- L1/LConn1
  Series RLC Branch3/RConn1 -- Full-Bridge MMC (External DC Links)/LConn2 -- Series RLC Branch1/RConn1
  Full-Bridge MMC (External DC Links)/RConn1 -- DC Voltage Source/RConn1
  Full-Bridge MMC (External DC Links)/RConn2 -- DC Voltage Source/LConn1
  Series RLC Branch/RConn1 -- Full-Bridge MMC (External DC Links)/LConn1
  Plasma_Load/RConn1 -- Current Measurement2/LConn1
  Series RLC Branch4/LConn1 -- Current Measurement2/RConn1
  L2/RConn1 -- Series RLC Branch3/LConn1
  Current Measurement/RConn1 -- L2/LConn1
  L1/RConn1 -- Current Measurement/LConn1 -- Voltage Measurement1/LConn1 -- C/LConn1
  Series RLC Branch1/LConn1 -- Voltage Measurement1/LConn2 -- C/RConn1

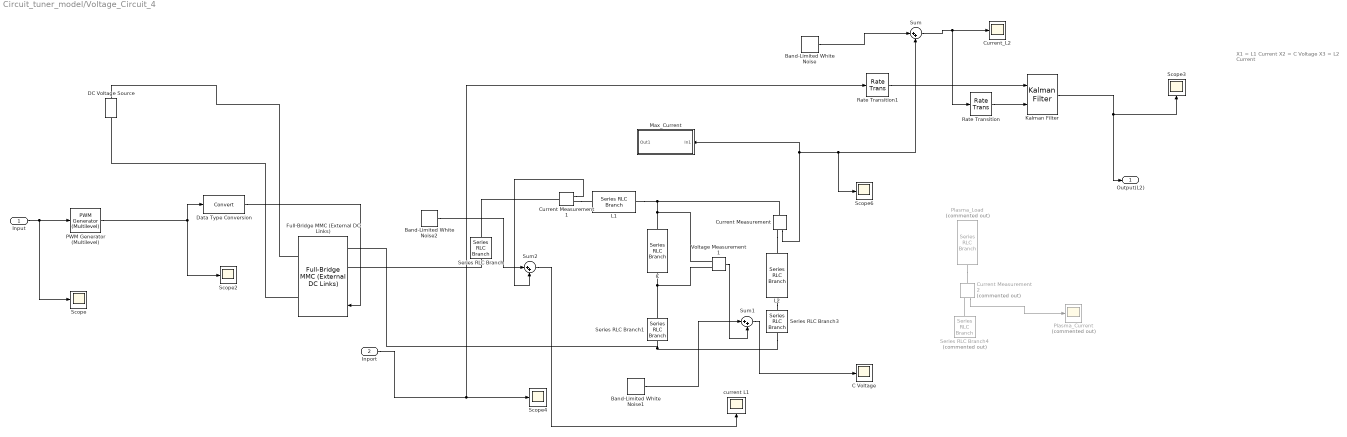
== system Circuit_tuner_model/Voltage_Circuit_4 ==
  note: X1 = L1 Current
      | X2 = C Voltage
      | X3 = L2 Current
  Input : Inport
  Inport : Inport  Port=2
  Band-Limited White Noise : simulink/Sources/Band-Limited White Noise  Cov=NoisePower  Ts=SampleTime  seed=[23341]
  Band-Limited White Noise1 : simulink/Sources/Band-Limited White Noise  Cov=NoisePower/5  Ts=SampleTime  seed=[23341]
  Band-Limited White Noise2 : simulink/Sources/Band-Limited White Noise  Cov=NoisePower  Ts=SampleTime  seed=[23341]
  C : spsSeriesRLCBranchLib/Series RLC Branch  LConnTagsString=__new0  RConnTagsString=__new0  BranchType=C  Resistance=1  Inductance=1e-3  SetiL0=off  InitialCurrent=0  Capacitance=Cap*2  Setx0=off  InitialVoltage=0  Measurements=None
  C Voltage : Scope
  Current Measurement : spsCurrentMeasurementLib/Current Measurement  PhasorSimulation=off  OutputType=Complex  PSBequivalent=0
  Current Measurement1 : spsCurrentMeasurementLib/Current Measurement  PhasorSimulation=off  OutputType=Complex  PSBequivalent=0
  Current Measurement2 : spsCurrentMeasurementLib/Current Measurement  Commented=on  PhasorSimulation=off  OutputType=Complex  PSBequivalent=0
  Current_L2 : Scope
  DC Voltage Source : spsDCVoltageSourceLib/DC Voltage Source  Amplitude=Amplitude  Measurements=None
  Data Type Conversion : DataTypeConversion  SaturateOnIntegerOverflow=off  RndMeth=Floor
  Full-Bridge MMC (External DC Links) : spsFullBridgeMMCExternalDCLinksLib/Full-Bridge MMC (External DC Links)  ModelType=Switching devices  n=1  Ron=1e-3  Rs=1e6  Cs=inf  Ron_Diode=1e-3  Rs_Diode=1e6  Cs_Diode=inf  Vf_Diode=1e-3  Rs_CurrentSource=inf  Ts=1e-6
      settings: SourceProductBaseCode=PS
  Kalman Filter : ctrlSharedLib/Kalman Filter  TimeDomain=Discrete-Time  UseCurrentEstimator=on  ModelSource=LTI State-Space Variable  ModelSourceVariable=sys_d  A=Ad  B=Bd  C=Cd  D=Dd  NumberOfStates=1  NumberOfInputs=1  NumberOfOutputs=1  InitialEstimateSource=Dialog  X0=voltage(1)  P0=10  UseK=off  UseGH=off  NumberOfProcessNoiseInputs=1  G=G  TimeInvariantG=on  H=0  TimeInvariantH=on  Q=Q  TimeInvariantQ=on  R=R  TimeInvariantR=on  N=0  TimeInvariantN=on  AddInputPort=on  AddEnablePort=off  OutputEstimatedY=off  OutputP=off  Ts=SampleTime
  L1 : spsSeriesRLCBranchLib/Series RLC Branch  LConnTagsString=__new0  RConnTagsString=__new0  BranchType=L  Resistance=1  Inductance=L1_V  SetiL0=off  InitialCurrent=0  Capacitance=0  Setx0=off  InitialVoltage=0  Measurements=None
  L2 : spsSeriesRLCBranchLib/Series RLC Branch  LConnTagsString=__new0  RConnTagsString=__new0  BranchType=L  Resistance=1  Inductance=L2  SetiL0=off  InitialCurrent=0  Capacitance=1e-6  Setx0=off  InitialVoltage=0  Measurements=None
  Max_Current : Subsystem
  PWM Generator (Multilevel) : spsPWMGeneratorMultilevelLib/PWM Generator (Multilevel)  BridgeType=Full-bridge  NumberOfBridges=1  Fc=1e3  Ts=0  ShowCarriersOutport=off
      settings: SourceProductBaseCode=PS
  Plasma_Current : Scope  Commented=on
  Plasma_Load : spsSeriesRLCBranchLib/Series RLC Branch  Commented=on  LConnTagsString=__new0  RConnTagsString=__new0  BranchType=L  Resistance=1  Inductance=Lp  SetiL0=off  InitialCurrent=0  Capacitance=1e-6  Setx0=off  InitialVoltage=0  Measurements=None
  Rate Transition : RateTransition
  Rate Transition1 : RateTransition
  Scope{,2..4,6} (5 alike) : Scope
  Series RLC Branch : spsSeriesRLCBranchLib/Series RLC Branch  LConnTagsString=__new0  RConnTagsString=__new0  BranchType=R  Resistance=R1  Inductance=1e-3  SetiL0=off  InitialCurrent=0  Capacitance=1e-6  Setx0=off  InitialVoltage=0  Measurements=None
  Series RLC Branch1 : spsSeriesRLCBranchLib/Series RLC Branch  LConnTagsString=__new0  RConnTagsString=__new0  BranchType=R  Resistance=R2  Inductance=1e-3  SetiL0=off  InitialCurrent=0  Capacitance=1e-6  Setx0=off  InitialVoltage=0  Measurements=None
  Series RLC Branch3 : spsSeriesRLCBranchLib/Series RLC Branch  LConnTagsString=__new0  RConnTagsString=__new0  BranchType=R  Resistance=R3  Inductance=1e-3  SetiL0=off  InitialCurrent=0  Capacitance=1e-6  Setx0=off  InitialVoltage=0  Measurements=None
  Series RLC Branch4 : spsSeriesRLCBranchLib/Series RLC Branch  Commented=on  LConnTagsString=__new0  RConnTagsString=__new0  BranchType=R  Resistance=.005  Inductance=1e-3  SetiL0=off  InitialCurrent=0  Capacitance=1e-6  Setx0=off  InitialVoltage=0  Measurements=None
  Sum : Sum  Inputs=|++
  Sum1 : Sum  Inputs=|++
  Sum2 : Sum  Inputs=|++
  Voltage Measurement1 : spsVoltageMeasurementLib/Voltage Measurement  PhasorSimulation=off  OutputType=Complex  PSBequivalent=0
  current L1 : Scope
  Output(L2) : Outport
  wires:
  Current Measurement1/1 -> Sum2/2
  PWM Generator (Multilevel)/1 -> Data Type Conversion/1, Scope2/1
  Input/1 -> Scope/1, PWM Generator (Multilevel)/1
  Current Measurement2/1 -> Plasma_Current/1
  Band-Limited White Noise/1 -> Sum/1
  Current Measurement/1 -> Max_Current/1(In1), Scope6/1, Sum/2
  Data Type Conversion/1 -> Full-Bridge MMC (External DC Links)/1
  Kalman Filter/1 -> Scope3/1, Output(L2)/1
  Sum2/1 -> current L1/1
  Band-Limited White Noise1/1 -> Sum1/1
  Voltage Measurement1/1 -> Sum1/2
  Band-Limited White Noise2/1 -> Sum2/1
  Sum1/1 -> C Voltage/1
  Sum/1 -> Rate Transition/1, Current_L2/1
  Inport/1 -> Rate Transition1/1, Scope4/1
  Rate Transition/1 -> Kalman Filter/2
  Rate Transition1/1 -> Kalman Filter/1
  connections:
  Current Measurement1/LConn1 -- Series RLC Branch/LConn1
  Current Measurement1/RConn1 -- L1/LConn1
  Series RLC Branch3/RConn1 -- Full-Bridge MMC (External DC Links)/LConn2 -- Series RLC Branch1/RConn1
  Full-Bridge MMC (External DC Links)/RConn1 -- DC Voltage Source/RConn1
  Full-Bridge MMC (External DC Links)/RConn2 -- DC Voltage Source/LConn1
  Series RLC Branch/RConn1 -- Full-Bridge MMC (External DC Links)/LConn1
  Plasma_Load/RConn1 -- Current Measurement2/LConn1
  Series RLC Branch4/LConn1 -- Current Measurement2/RConn1
  L2/RConn1 -- Series RLC Branch3/LConn1
  Current Measurement/RConn1 -- L2/LConn1
  L1/RConn1 -- Current Measurement/LConn1 -- Voltage Measurement1/LConn1 -- C/LConn1
  Series RLC Branch1/LConn1 -- Voltage Measurement1/LConn2 -- C/RConn1

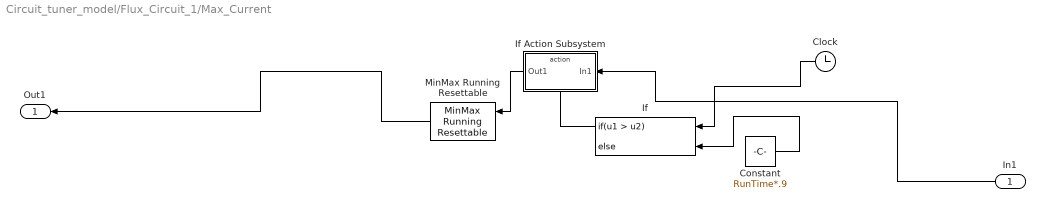
== system Circuit_tuner_model/Flux_Circuit_1/Max_Current ==
  In1 : Inport
  Clock : Clock
  Constant : Constant  Value=RunTime*.9
  If : If  NumInputs=2  IfExpression=u1 > u2
  If Action Subsystem : Subsystem  TreatAsAtomicUnit=on
  MinMax Running Resettable : simulink/Math Operations/MinMax Running Resettable  Function=max  vinit=0.0
  Out1 : Outport
  wires:
  In1/1 -> If Action Subsystem/1(In1)
  If Action Subsystem/1(Out1) -> MinMax Running Resettable/1
  MinMax Running Resettable/1 -> Out1/1
  Constant/1 -> If/2
  Clock/1 -> If/1
  If/1 -> If Action Subsystem/Action
